simulink model "stc"  (R2018b)
settings: Solver=FixedStepDiscrete  StartTime=0.0  StopTime=0.49  RelTol=1e-3
PreLoadFcn:
  | load mtlb;
  | load candidatePitch;
undefined symbols (not defined in the file or in its folder): mtlb
libraries: dspsigops x3, dsplp x2, dspsrcs4 x1, dspspect3 x1, dspsolvers x1
settings Model: Creator=paulochiliguano  LastModifiedBy=usuario
settings ConfigComp: DVTestSuiteOptimization=CombinedObjectives (Nonlinear Extended)  DVDetectOutOfBounds=on

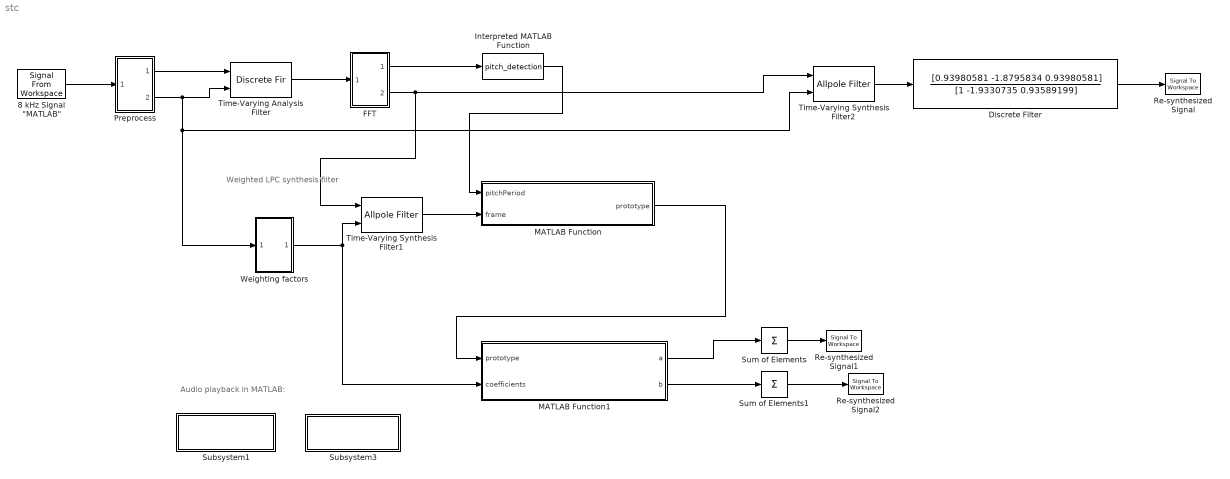
== system stc ==
  note: Weighted LPC synthesis filter
  note: Audio playback in MATLAB:
  "8 kHz Signal \"MATLAB\"" : dspsrcs4/Signal From Workspace  X=mtlb*0.5  Ts=1/8000  nsamps=80  OutputAfterFinalValue=Setting to zero  ignoreOrWarnInputAndFrameLengths=off  OutputFrames=off
  Discrete Filter : DiscreteFilter  Numerator=[0.93980581 -1.8795834 0.93980581]  Denominator=[1 -1.9330735 0.93589199]  InputProcessing=Columns as channels (frame based)  FilterStructure=Direct form II transposed  a0EqualsOne=on
  FFT : Subsystem
  Interpreted MATLAB Function : MATLABFcn  MATLABFcn=pitch_detection
  MATLAB Function : MATLAB Function  TreatAsAtomicUnit=on
  MATLAB Function1 : MATLAB Function  TreatAsAtomicUnit=on
  Preprocess : Subsystem
  Re-synthesized Signal : SignalToWorkspace  VariableName=y_stc
  Re-synthesized Signal1 : SignalToWorkspace  VariableName=y_stc1
  Re-synthesized Signal2 : SignalToWorkspace  VariableName=y_stc2
  Subsystem1 : Subsystem
      settings: OpenFcn=if exist('mtlb','var'), sound(mtlb*0.32,8000); else errordlg('Data not found in workspace - reload demo model.','DSP Blockset Demo Error'); end
      mask Display: disp('Original\nSignal')
  Subsystem3 : Subsystem
      settings: OpenFcn=if exist('y_stc','var'), sound(y_stc,8000); else errordlg('You must run the simulation first.','DSP Blockset Demo Error'); end
      mask Display: disp('Processed\nSignal')
  Sum of Elements : Sum  Inputs=+
  Sum of Elements1 : Sum  Inputs=+
  Time-Varying Analysis Filter : DiscreteFir  CoefSource=Input port  Coefficients=[0.2 0.4]  InputProcessing=Columns as channels (frame based)  AccumDataTypeStr=Inherit: Same as product output  OutDataTypeStr=Inherit: Same as input
      settings: InputPortMap=u0,u1
  Time-Varying Synthesis Filter1 : AllpoleFilter  CoefSource=Input port  Coefficients=[0.2 0.4]  AccumDataTypeStr=Inherit: Same as product output
      settings: InputPortMap=u0,u1
  Time-Varying Synthesis Filter2 : AllpoleFilter  CoefSource=Input port  Coefficients=[0.2 0.4]  AccumDataTypeStr=Inherit: Same as product output
      settings: InputPortMap=u0,u1
  Weighting factors : Subsystem
  wires:
  Interpreted MATLAB Function/1 -> MATLAB Function/1(pitchPeriod)
  Discrete Filter/1 -> Re-synthesized Signal/1
  "8 kHz Signal \"MATLAB\""/1 -> Preprocess/1(In1)
  Preprocess/1(Out1) -> Time-Varying Analysis Filter/1
  Time-Varying Synthesis Filter1/1 -> MATLAB Function/2(frame)
  Preprocess/2(Out2) -> Time-Varying Analysis Filter/2, Time-Varying Synthesis Filter2/2, Weighting factors/1(In1)
  MATLAB Function1/1(a) -> Sum of Elements/1
  MATLAB Function1/2(b) -> Sum of Elements1/1
  Sum of Elements1/1 -> Re-synthesized Signal2/1
  Sum of Elements/1 -> Re-synthesized Signal1/1
  Time-Varying Analysis Filter/1 -> FFT/1(In1)
  FFT/1(Out1) -> Interpreted MATLAB Function/1
  MATLAB Function/1(prototype) -> MATLAB Function1/1(prototype)
  Weighting factors/1(Out1) -> MATLAB Function1/2(coefficients), Time-Varying Synthesis Filter1/2
  FFT/2(Out2) -> Time-Varying Synthesis Filter1/1, Time-Varying Synthesis Filter2/1
  Time-Varying Synthesis Filter2/1 -> Discrete Filter/1

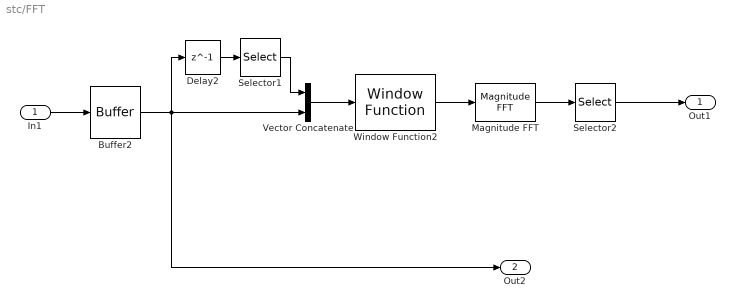
== system stc/FFT ==
  In1 : Inport
  Buffer2 : Buffer  N=160  OutputFrames=off
  Delay2 : Delay  DelayLength=1  InputProcessing=Inherited
  Magnitude FFT : dspspect3/Magnitude FFT  mag_or_magsq=Magnitude  FFTImplementation=Auto  fftLenInherit=off  fftsize=512  WrapInput=on
      settings: SourceProductName=DSP System Toolbox  SourceProductBaseCode=DS
  Selector1 : Selector  IndexOptions=Starting index (dialog)  Indices=81  OutputSizes=80
  Selector2 : Selector  IndexOptions=Starting index (dialog)  Indices=1  OutputSizes=65
  Vector Concatenate : Concatenate
  Window Function2 : dspsigops/Window Function  winmode=Apply window to input  wintype=Hamming  sampmode=Continuous  samptime=1  N=64  Rs=50  beta=10  winsamp=Symmetric  UserWindow=hamming  OptParams=off  UserParams={'symmetric'}  dataType=double  isSigned=on  wordLen=16  udDataType=sfix(16)  fracBitsMode=Best precision  numFracBits=15  roundingMode=Floor  overflowMode=off  numSidelobes=4  sidelobeLevel=-30
      settings: SourceProductName=DSP System Toolbox  SourceProductBaseCode=DS
  Out1 : Outport
  Out2 : Outport  Port=2
  wires:
  Window Function2/1 -> Magnitude FFT/1
  Selector1/1 -> Vector Concatenate/1
  Buffer2/1 -> Out2/1, Vector Concatenate/2, Delay2/1
  Vector Concatenate/1 -> Window Function2/1
  Magnitude FFT/1 -> Selector2/1
  In1/1 -> Buffer2/1
  Delay2/1 -> Selector1/1
  Selector2/1 -> Out1/1

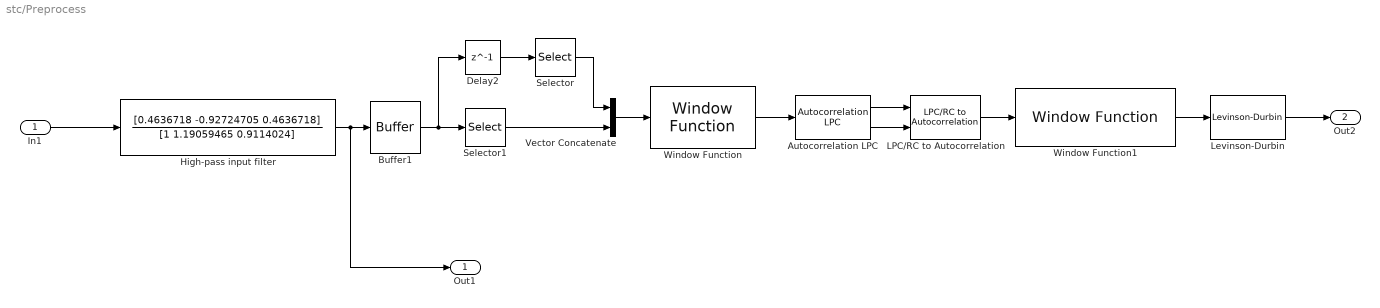
== system stc/Preprocess ==
  In1 : Inport
  Autocorrelation LPC : dsplp/Autocorrelation LPC  lpcCoeffOutFcn=A  lpcOutP=on  inherit_prediction_order=off  order=10
      settings: SourceProductName=DSP System Toolbox  SourceProductBaseCode=DS
  Buffer1 : Buffer  N=160  OutputFrames=off
  Delay2 : Delay  DelayLength=1  InputProcessing=Inherited
  High-pass input filter : DiscreteFilter  Numerator=[0.4636718 -0.92724705 0.4636718]  Denominator=[1 1.19059465 0.9114024]  InputProcessing=Columns as channels (frame based)  FilterStructure=Direct form II transposed  a0EqualsOne=on
  LPC/RC to Autocorrelation : dsplp/LPC//RC to Autocorrelation  conversion=LPC to autocorrelation  perr_spec=Via input port  error=Replace it with 1
      settings: SourceProductName=DSP System Toolbox  SourceProductBaseCode=DS
  Levinson-Durbin : dspsolvers/Levinson-Durbin  coeffOutFcn=OBSOLETE  coeffOutFcnActive=A  outP=off  zeroInpHandling=on  roundingMode=Floor  overflowMode=off  prodOutputMode=User-defined  prodOutputWordLength=32  prodOutputFracLength=30  prodOutputDataTypeStr=fixdt(1,32,30)  prodOutputLastDataTypeStr=fixdt(1,32,30)  accumMode=User-defined  accumWordLength=32  accumFracLength=30  accumDataTypeStr=fixdt(1,32,30)  accumLastDataTypeStr=fixdt(1,32,30)  firstCoeffMode=Binary point scaling  firstCoeffWordLength=16  firstCoeffFracLength=15  firstCoeffDataTypeStr=fixdt(1,16,15)  firstCoeffMin=[]  firstCoeffMax=[]  firstCoeffLastDataTypeStr=fixdt(1,16,15)  secondCoeffMode=Binary point scaling  secondCoeffWordLength=16  secondCoeffFracLength=15  secondCoeffDataTypeStr=fixdt(1,16,15)  secondCoeffMin=[]  secondCoeffMax=[]  secondCoeffLastDataTypeStr=fixdt(1,16,15)  outputMin=[]  outputMax=[]
      settings: SourceProductName=DSP System Toolbox  SourceProductBaseCode=DS  allowOverrides=off
  Selector : Selector  IndexOptions=Starting index (dialog)  Indices=41  OutputSizes=120
  Selector1 : Selector  IndexOptions=Starting index (dialog)  Indices=1  OutputSizes=120
  Vector Concatenate : Concatenate
  Window Function : dspsigops/Window Function  winmode=Apply window to input  wintype=User defined  sampmode=Continuous  samptime=1  N=64  Rs=50  beta=10  winsamp=Symmetric  UserWindow=hybrid_window  OptParams=off  UserParams={'symmetric'}  dataType=double  isSigned=on  wordLen=16  udDataType=sfix(16)  fracBitsMode=Best precision  numFracBits=15  roundingMode=Floor  overflowMode=off  numSidelobes=4  sidelobeLevel=-30
      settings: SourceProductName=DSP System Toolbox  SourceProductBaseCode=DS
  Window Function1 : dspsigops/Window Function  winmode=Apply window to input  wintype=User defined  sampmode=Continuous  samptime=1  N=64  Rs=50  beta=10  winsamp=Symmetric  UserWindow=bandwidth_expansion  OptParams=off  UserParams={'symmetric'}  dataType=double  isSigned=on  wordLen=16  udDataType=sfix(16)  fracBitsMode=Best precision  numFracBits=15  roundingMode=Floor  overflowMode=off  numSidelobes=4  sidelobeLevel=-30
      settings: SourceProductName=DSP System Toolbox  SourceProductBaseCode=DS
  Out1 : Outport
  Out2 : Outport  Port=2
  wires:
  Window Function/1 -> Autocorrelation LPC/1
  Buffer1/1 -> Selector1/1, Delay2/1
  Autocorrelation LPC/2 -> LPC/RC to Autocorrelation/2
  Delay2/1 -> Selector/1
  High-pass input filter/1 -> Out1/1, Buffer1/1
  LPC/RC to Autocorrelation/1 -> Window Function1/1
  Selector1/1 -> Vector Concatenate/2
  Selector/1 -> Vector Concatenate/1
  Autocorrelation LPC/1 -> LPC/RC to Autocorrelation/1
  Vector Concatenate/1 -> Window Function/1
  Window Function1/1 -> Levinson-Durbin/1
  In1/1 -> High-pass input filter/1
  Levinson-Durbin/1 -> Out2/1

== system stc/Subsystem1 ==

== system stc/Subsystem3 ==

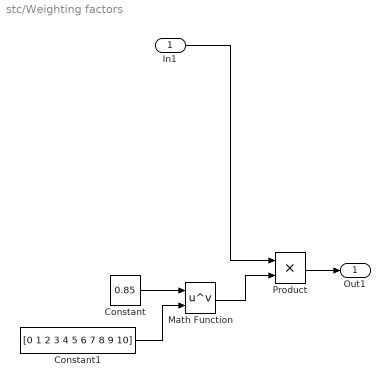
== system stc/Weighting factors ==
  In1 : Inport
  Constant : Constant  Value=0.85
  Constant1 : Constant  Value=[0 1 2 3 4 5 6 7 8 9 10]
  Math Function : Math  Operator=pow  SaturateOnIntegerOverflow=on
  Product : Product
  Out1 : Outport
  wires:
  In1/1 -> Product/1
  Constant/1 -> Math Function/1
  Constant1/1 -> Math Function/2
  Math Function/1 -> Product/2
  Product/1 -> Out1/1

== matlab function stc/MATLAB Function1 ==
  data: prototype input; a output size=80; coefficients input; b output size=80
function [a, b] = sinusoidal_coefficients(prototype, coefficients)
%
% Name: Paulo Esteban Chiliguano Torres
% Date: 2018/11/21
% Revision: 1.0

% Prototype length
P = length(prototype);
N = P;
disp(coefficients)

% Error signal DFT
Ek = fft(prototype);
real_Ek = real(Ek(1:ceil(P/2)));
imag_Ek = imag(Ek(1:ceil(P/2)));

% Weighted LPC synthesis filter impulse response
imp = [1; zeros(P-1,1)];
[h, ~] = filter(1,coefficients,imp);

% Impulse response DFT
H = fft(h);
real_H = real(H(1:ceil(P/2)));
imag_H = imag(H(1:ceil(P/2)));

% George and Smith definitions
psi1 = real_Ek .* real_H + imag_Ek .* imag_H;
psi2 = real_Ek .* imag_H - imag_Ek .* real_H;
gamma11 = N/2 * real_H.^2 + N/2 * imag_H.^2;
gamma22 = gamma11;
%gamma12 = 0; % no longer needed

% a, b coefficients
a = psi1./gamma11;
b = psi2./gamma22;

% Amplitudes
%amplitudes = sqrt(a.^2 + b.^2);

% Phases
%phases = -atan(b./a);
end

== matlab function stc/MATLAB Function ==
  data: pitchPeriod input; frame input; prototype output size=147
function prototype  = select_prototype(pitchPeriod, frame)
%
% Name: Paulo Esteban Chiliguano Torres
% Date: 2018/11/21
% Revision: 1.0

% Frame length
FL = length(frame);

% Initial prototype selection
a = FL/2+1-round(pitchPeriod/2);
b = pitchPeriod+a-1;

% Maximum amplitude of the frame
[~, I] = max(frame(a:b));
max_frame = I+a-1;

%
if max_frame+pitchPeriod-1 <= FL
    a = max_frame;
end

% Zero-crossing
for j = a:-1:2
    if frame(j)>0 && frame(j-1)<=0
        if abs(frame(j)) < abs(frame(j-1))
            a = j;
        elseif abs(frame(j-1)) < abs(frame(j))
            a = j-1;
        end
        break;
    end
end

% Prototype waveform
prototype = frame(a:b);
end
